simulink model "HighLevel"  (R2023b)
settings: Solver=VariableStepAuto  StartTime=0.0  StopTime=1000  RelTol=1e-3
undefined symbols (not defined in the file or in its folder): DiscIntNeverNeededParam
libraries: simulink x6
settings Model: SimulationMode=accelerator  Creator=schro  LastModifiedBy=ijifl
settings DebuggingCC: AlgebraicLoopMsg=none

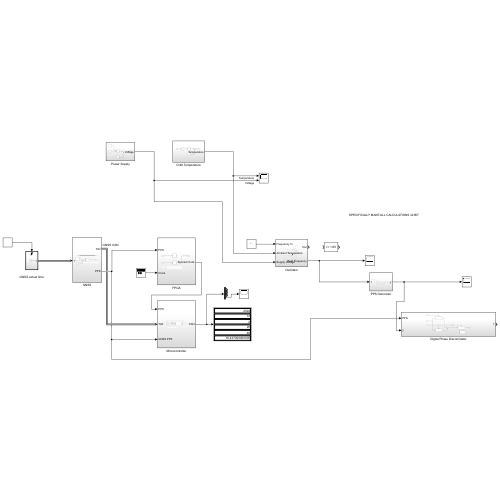
[thumbnail: Simulink's stored preview of the top-level diagram]
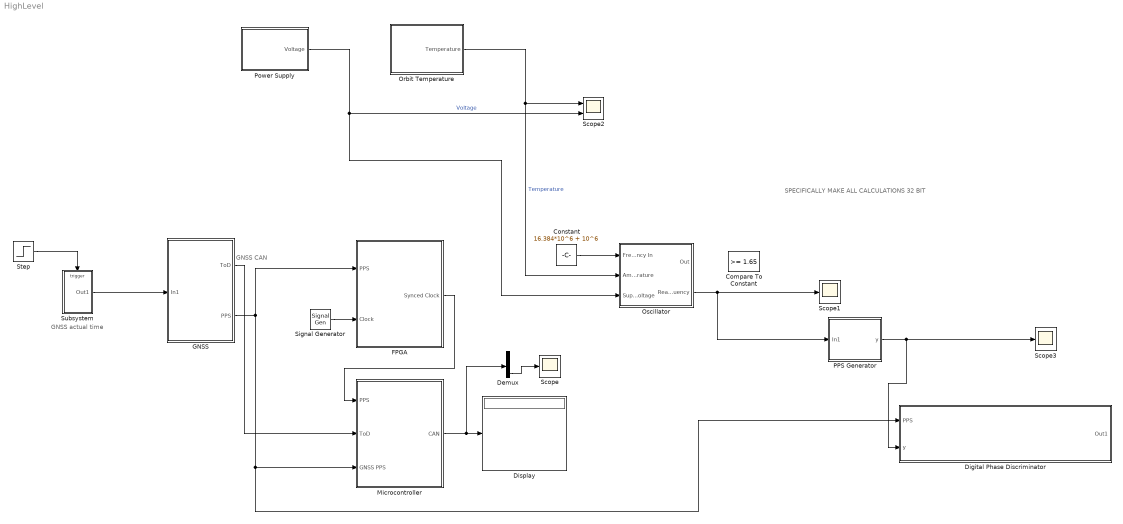
== system HighLevel ==
  note: SPECIFICALLY MAKE ALL CALCULATIONS 32 BIT
  note: GNSS CAN
  note: GNSS actual time
  Compare To Constant : simulink/Logic and Bit Operations/Compare To Constant  relop=>=  const=1.65  OutDataTypeStr=boolean
  Constant : Constant  Value=16.384*10^6 + 10^6
  Demux : Demux  Outputs=6
  Digital Phase Discriminator : Subsystem
  Display : Display
      settings: Format=decimal (Stored Integer)
  FPGA : Subsystem
  GNSS : Subsystem
  Microcontroller : Subsystem
  Orbit Temperature : Subsystem
  Oscillator : Subsystem
  PPS Generator : Subsystem
  Power Supply : Subsystem
  Scope : Scope
  Scope1 : Scope
  Scope2 : Scope  NumInputPorts=2
  Scope3 : Scope
  Signal Generator : SignalGenerator  WaveForm=square
  Step : Step  SampleTime=0
  Subsystem : Subsystem
  wires:
  GNSS/2(PPS) -> Digital Phase Discriminator/1(PPS), Microcontroller/3(GNSS PPS), FPGA/1(PPS)
  Signal Generator/1 -> FPGA/2(Clock)
  Subsystem/1(Out1) -> GNSS/1(In1)
  Step/1 -> Subsystem/Trigger
  Demux/6 -> Scope/1
  Microcontroller/1(CAN) -> Demux/1, Display/1
  FPGA/1(Synced Clock) -> Microcontroller/1(PPS)
  GNSS/1(ToD) -> Microcontroller/2(ToD)
  Constant/1 -> Oscillator/1(Frequency In)
  Orbit Temperature/1(Temperature) -> Scope2/1, Oscillator/2(Ambient Temperature)  "Temperature"
  Power Supply/1(Voltage) -> Scope2/2, Oscillator/3(Supply Voltage)  "Voltage"
  Oscillator/2(Real Frequency) -> PPS Generator/1(In1), Scope1/1
  PPS Generator/1(y) -> Digital Phase Discriminator/2(y), Scope3/1

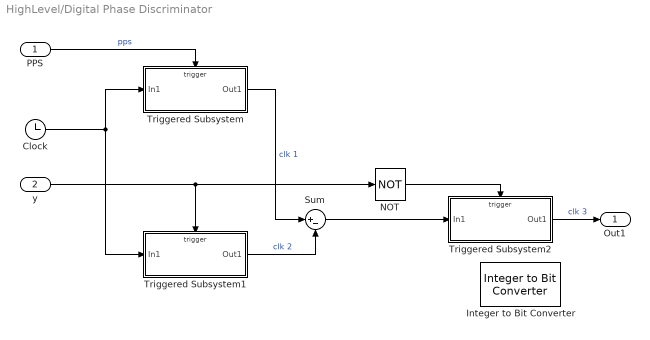
== system HighLevel/Digital Phase Discriminator ==
  PPS : Inport
  y : Inport  Port=2
  Clock : Clock
  Integer to Bit Converter : simulink/Logic and Bit Operations/Integer to Bit Converter  nbits=3  signedInputValues=Unsigned  bitOrder=MSB first  outDtype=Inherit via internal rule
  NOT : Logic  Operator=NOT  IconShape=distinctive  AllPortsSameDT=off  OutDataTypeStr=boolean
  Sum : Sum  Inputs=|+-
  Triggered Subsystem : Subsystem  TreatAsAtomicUnit=on
  Triggered Subsystem1 : Subsystem  TreatAsAtomicUnit=on
  Triggered Subsystem2 : Subsystem  TreatAsAtomicUnit=on
  Out1 : Outport
  wires:
  Triggered Subsystem/1(Out1) -> Sum/1  "clk 1"
  Clock/1 -> Triggered Subsystem/1(In1), Triggered Subsystem1/1(In1)
  NOT/1 -> Triggered Subsystem2/Trigger
  Triggered Subsystem1/1(Out1) -> Sum/2  "clk 2"
  Sum/1 -> Triggered Subsystem2/1(In1)
  Triggered Subsystem2/1(Out1) -> Out1/1  "clk 3"
  y/1 -> Triggered Subsystem1/Trigger, NOT/1
  PPS/1 -> Triggered Subsystem/Trigger  "pps"

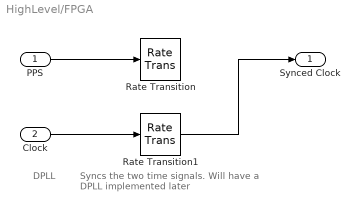
== system HighLevel/FPGA ==
  note: Syncs the two time signals.
      | Will have a DPLL implemented later
  note: DPLL
  PPS : Inport
  Clock : Inport  Port=2
  Rate Transition : RateTransition
  Rate Transition1 : RateTransition
  Synced Clock : Outport
  wires:
  PPS/1 -> Rate Transition/1
  Clock/1 -> Rate Transition1/1
  Rate Transition1/1 -> Synced Clock/1

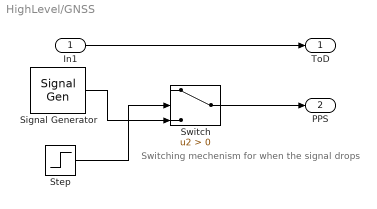
== system HighLevel/GNSS ==
  note: Switching mechenism for when the signal drops
  In1 : Inport
  Signal Generator : SignalGenerator  WaveForm=square
  Step : Step  Time=100000  SampleTime=0
  Switch : Switch  Criteria=u2 > Threshold  SaturateOnIntegerOverflow=off  InputSameDT=off
  ToD : Outport
  PPS : Outport  Port=2
  wires:
  In1/1 -> ToD/1
  Switch/1 -> PPS/1
  Step/1 -> Switch/2
  Signal Generator/1 -> Switch/3

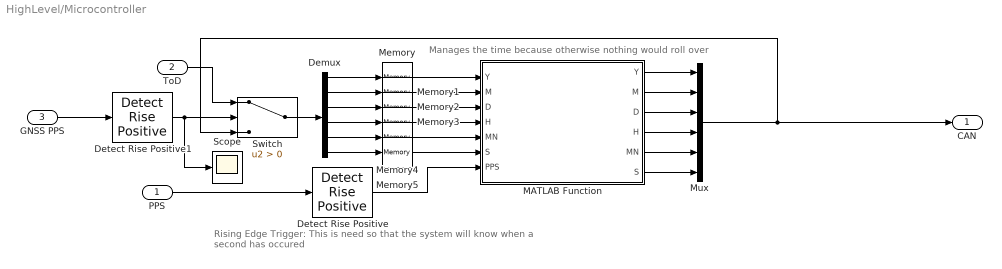
== system HighLevel/Microcontroller ==
  note: Manages the time because otherwise nothing would roll over
  note: Rising Edge Trigger:
      | This is need so that the system will know when a second has occured
  PPS : Inport
  ToD : Inport  Port=2
  GNSS PPS : Inport  Port=3
  Demux : Demux  Outputs=6
  Detect Rise Positive : simulink/Logic and Bit Operations/Detect Rise Positive  vinit=0  OutDataTypeStr=boolean
  Detect Rise Positive1 : simulink/Logic and Bit Operations/Detect Rise Positive  vinit=0  OutDataTypeStr=boolean
  MATLAB Function : MATLAB Function  TreatAsAtomicUnit=on
  Memory{,1..5} (6 alike) : Memory
  Mux : Mux  Inputs=6
  Scope : Scope
  Switch : Switch  Criteria=u2 > Threshold  SaturateOnIntegerOverflow=off  InputSameDT=off
  CAN : Outport
  wires:
  MATLAB Function/6(S) -> Mux/6
  MATLAB Function/5(MN) -> Mux/5
  MATLAB Function/4(H) -> Mux/4
  MATLAB Function/2(M) -> Mux/2
  MATLAB Function/3(D) -> Mux/3
  MATLAB Function/1(Y) -> Mux/1
  Detect Rise Positive/1 -> MATLAB Function/7(PPS)
  Mux/1 -> Switch/3, CAN/1
  PPS/1 -> Detect Rise Positive/1
  Switch/1 -> Demux/1
  ToD/1 -> Switch/1
  Detect Rise Positive1/1 -> Scope/1, Switch/2
  GNSS PPS/1 -> Detect Rise Positive1/1
  Demux/1 -> Memory/1
  Memory/1 -> MATLAB Function/1("Y ")
  Demux/2 -> Memory1/1
  Memory1/1 -> MATLAB Function/2("M ")
  Demux/3 -> Memory2/1
  Memory2/1 -> MATLAB Function/3("D ")
  Demux/4 -> Memory3/1
  Memory3/1 -> MATLAB Function/4("H ")
  Demux/6 -> Memory5/1
  Demux/5 -> Memory4/1
  Memory5/1 -> MATLAB Function/6("S ")
  Memory4/1 -> MATLAB Function/5("MN ")

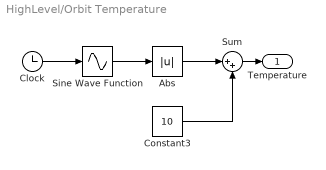
== system HighLevel/Orbit Temperature ==
  Abs : Abs  SaturateOnIntegerOverflow=off
  Clock : Clock
  Constant3 : Constant  Value=10
  Sine Wave Function : Sin  TimeSource=Use external signal  Amplitude=11  Frequency=2*pi*8/(24*60*60)  SampleTime=0
  Sum : Sum  Inputs=|++
  Temperature : Outport
  wires:
  Constant3/1 -> Sum/2
  Sine Wave Function/1 -> Abs/1
  Abs/1 -> Sum/1
  Sum/1 -> Temperature/1
  Clock/1 -> Sine Wave Function/1

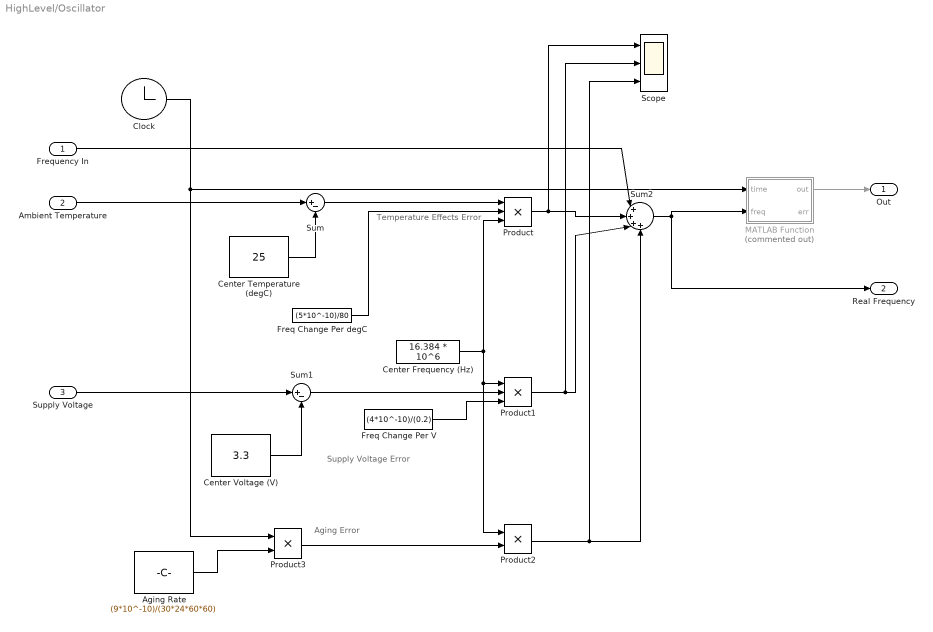
== system HighLevel/Oscillator ==
  note: Temperature Effects Error
  note: Supply Voltage Error
  note: Aging Error
  Frequency In : Inport
  Ambient Temperature : Inport  Port=2
  Supply Voltage : Inport  Port=3
  Aging Rate : Constant  Value=(9*10^-10)/(30*24*60*60)
  Center Frequency (Hz) : Constant  Value=16.384 * 10^6
  Center Temperature (degC) : Constant  Value=25
  Center Voltage (V) : Constant  Value=3.3
  Clock : Clock
  Freq Change Per V : Constant  Value=(4*10^-10)/(0.2)
  Freq Change Per degC : Constant  Value=(5*10^-10)/80
  MATLAB Function : MATLAB Function  Commented=on  TreatAsAtomicUnit=on
  Product : Product  Inputs=3
  Product1 : Product  Inputs=3
  Product2 : Product
  Product3 : Product
  Scope : Scope  NumInputPorts=3
  Sum : Sum  Inputs=|+-
  Sum1 : Sum  Inputs=|+-
  Sum2 : Sum  Inputs=|++++
  Out : Outport
  Real Frequency : Outport  Port=2
  wires:
  Frequency In/1 -> Sum2/1
  MATLAB Function/1(out) -> Out/1
  Clock/1 -> Product3/1, MATLAB Function/1(time)
  Ambient Temperature/1 -> Sum/1
  Center Temperature (degC)/1 -> Sum/2
  Sum/1 -> Product/1
  Freq Change Per degC/1 -> Product/2
  Sum1/1 -> Product1/2
  Supply Voltage/1 -> Sum1/1
  Center Voltage (V)/1 -> Sum1/2
  Freq Change Per V/1 -> Product1/3
  Product/1 -> Scope/1, Sum2/2
  Product1/1 -> Scope/2, Sum2/3
  Sum2/1 -> Real Frequency/1, MATLAB Function/2(freq)
  Product2/1 -> Scope/3, Sum2/4
  Product3/1 -> Product2/2
  Aging Rate/1 -> Product3/2
  Center Frequency (Hz)/1 -> Product/3, Product2/1, Product1/1

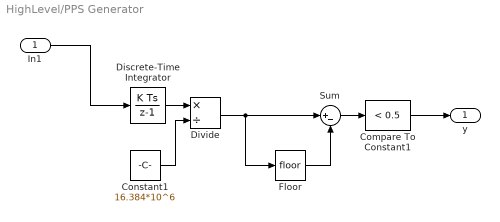
== system HighLevel/PPS Generator ==
  In1 : Inport
  Compare To Constant1 : simulink/Logic and Bit Operations/Compare To Constant  relop=<  const=0.5  OutDataTypeStr=boolean
  Constant1 : Constant  Value=16.384*10^6
  Discrete-Time Integrator : DiscreteIntegrator  SampleTime=-1  ICPrevOutput=DiscIntNeverNeededParam  ICPrevScaledInput=DiscIntNeverNeededParam
  Divide : Product  Inputs=*/
  Floor : Rounding
  Sum : Sum  Inputs=|+-
  y : Outport
  wires:
  Discrete-Time Integrator/1 -> Divide/1
  Constant1/1 -> Divide/2
  Divide/1 -> Floor/1, Sum/1
  Floor/1 -> Sum/2
  In1/1 -> Discrete-Time Integrator/1
  Sum/1 -> Compare To Constant1/1
  Compare To Constant1/1 -> y/1

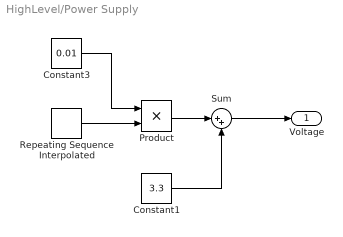
== system HighLevel/Power Supply ==
  Constant1 : Constant  Value=3.3
  Constant3 : Constant  Value=0.01
  Product : Product
  Repeating Sequence Interpolated : simulink/Sources/Repeating Sequence Interpolated  OutValues=[0 1 0].'  TimeValues=[0 0.1 0.2].'  LookUpMeth=Interpolation-Use End Values  tsamp=0.01  OutMin=[]  OutMax=[]  OutDataTypeStr=double  OutputDataTypeScalingMode=double  OutDataType=fixdt(0,8)  OutScaling=2^-10
  Sum : Sum  Inputs=|++
  Voltage : Outport
  wires:
  Constant1/1 -> Sum/2
  Product/1 -> Sum/1
  Constant3/1 -> Product/1
  Repeating Sequence Interpolated/1 -> Product/2
  Sum/1 -> Voltage/1

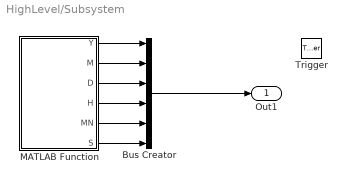
== system HighLevel/Subsystem ==
  Trigger : TriggerPort  VariantControl=(inherit)  PortDimensions=1
  Bus Creator : BusCreator  Inputs=6
  MATLAB Function : MATLAB Function  TreatAsAtomicUnit=on
  Out1 : Outport
  wires:
  Bus Creator/1 -> Out1/1
  MATLAB Function/1(Y) -> Bus Creator/1
  MATLAB Function/2(M) -> Bus Creator/2
  MATLAB Function/4(H) -> Bus Creator/4
  MATLAB Function/3(D) -> Bus Creator/3
  MATLAB Function/6(S) -> Bus Creator/6
  MATLAB Function/5(MN) -> Bus Creator/5

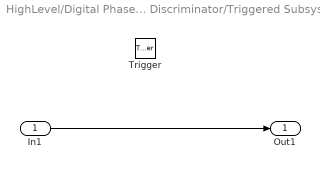
== system HighLevel/Digital Phase Discriminator/Triggered Subsystem ==
  In1 : Inport
  Trigger : TriggerPort  VariantControl=(inherit)
  Out1 : Outport
  wires:
  In1/1 -> Out1/1

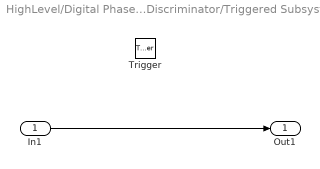
== system HighLevel/Digital Phase Discriminator/Triggered Subsystem1 ==
  In1 : Inport
  Trigger : TriggerPort  VariantControl=(inherit)
  Out1 : Outport
  wires:
  In1/1 -> Out1/1

== system HighLevel/Digital Phase Discriminator/Triggered Subsystem2 ==
  In1 : Inport
  Trigger : TriggerPort  VariantControl=(inherit)
  Out1 : Outport
  wires:
  In1/1 -> Out1/1

== matlab function HighLevel/Microcontroller/MATLAB Function ==
  data: Y input; Y output; M input; D input; H input; MN input; S input; PPS input; M output; D output; H output; MN output; S output
function [Y, M, D, H, MN, S] = TimeKeeping(Y, M, D, H, MN, S, PPS)
   
   if (PPS == 1)
       S = S + 1;
   end
   if (S > 60)
       S = S- 60;
       MN = MN+1;
   end
   if (MN > 60)
       MN = MN - 60;
       H = H + 1;
   end
   if (H > 24)
       H = H - 24;
       D = D + 1;
   end
   if (D > 30)
       D = D - 30;
       M = M + 1;
   end
   if (M > 12)
       M = M - 12;
       Y = Y+1;
   end
end

== matlab function HighLevel/Subsystem/MATLAB Function ==
  data: Y output; M output; D output; H output; MN output; S output
function [Y, M, D, H, MN, S] = fcn()
   eml.extrinsic('now');
   eml.extrinsic('datevec');
   Y = 0;
   M = 0;
   D = 0;
   H = 0;
   MN = 0;
   S = 0;
   [Y, M, D, H, MN, S] = datevec(now);
end

== matlab function HighLevel/Oscillator/MATLAB Function ==
  data: time input; freq input; out output; err output
function [out,err] = fcn(time, freq)
    out = 1.65*sin(2*pi*time*freq) + 1.65;
    err = 0;
end
